simulink model "longSimworks"  (R2023a)
settings: Solver=VariableStepAuto  StartTime=0.0  StopTime=30  RelTol=1e-3
settings Model: Creator=User  LastModifiedBy=User

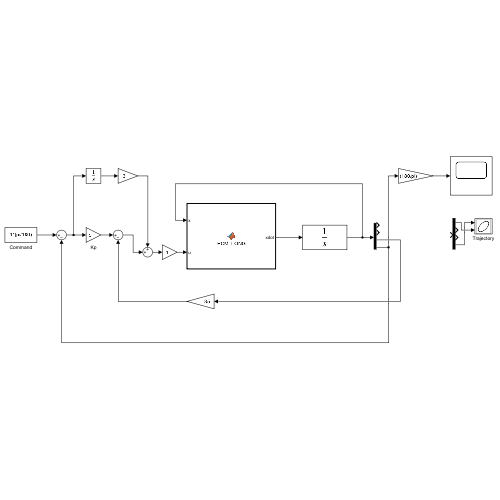
[thumbnail: Simulink's stored preview of the top-level diagram]
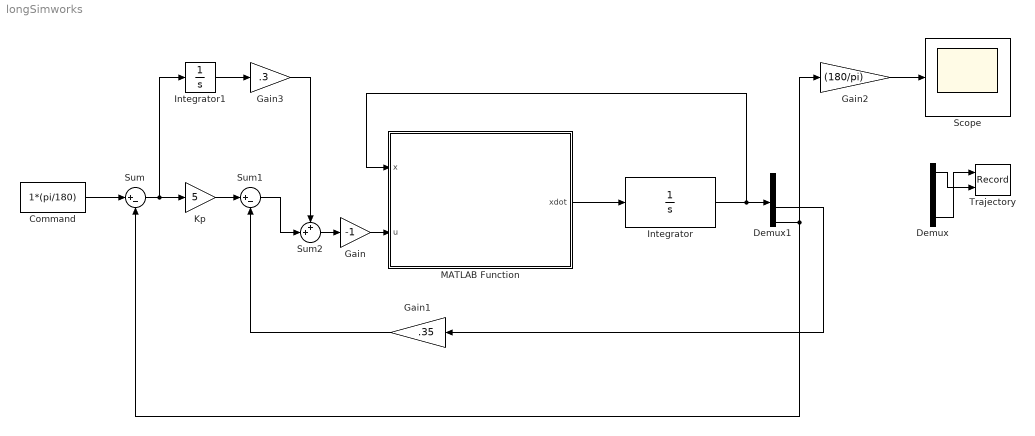
== system longSimworks ==
  Command : Constant  Value=1*(pi/180)
  Demux : Demux
  Demux1 : Demux
  Gain : Gain  Gain=-1
  Gain1 : Gain  Gain=.35
  Gain2 : Gain  Gain=(180/pi)
  Gain3 : Gain  Gain=.3
  Integrator : Integrator  InitialCondition=[0; 0; 0; 0]
  Integrator1 : Integrator
  Kp : Gain  Gain=5
  MATLAB Function : MATLAB Function  TreatAsAtomicUnit=on
  Scope : Scope
  Sum : Sum  Inputs=|+-
  Sum1 : Sum  Inputs=|+-
  Sum2 : Sum  Inputs=++|
  Trajectory : Record  FileSettingsInternal="{\"entries\":[{\"content\":{\"excelSettings\":{\"content\":{},\"type\":\"Streamout.ExcelSettings\"}},\"type\":\"Streamout.FileSettingStorage\",\"uuid\":\"55440844-dddf-4c7d-848c-ec0167b170e0\"}],\"packageUris\":[\"http://schema.mathworks.com/mf0/streamout_blocks/R2020a\"],\"version\":\"1.0\"}"  Layout=[1 2]  SignalsInternal="{\"entries\":[{\"content\":{\"signals\":[{\"content\":{\"blockPath\":[\"longSimworks/Trajectory\"],\"dimensions\":[1],\"domain\":\"longSimworks/Trajectory\",\"lineColor\":\"#a2142f\",\"plots\":[1],\"port\":1,\"sid\":[\"\"],\"signalID\":205,\"signalName\":\"Demux:4\"},\"type\":\"RecordBlkView.Signal\",\"uuid\":\"3001cd2d-3298-47da-9ba3-97cff598d7e7\"},{\"content\":{\"blockPath\":[\"longSimworks/Trajectory\"],\"dimensions\":[1],\"domain\":\"longSimworks/Trajectory\",\"lineColor\":\"#139fff\",\"plots\":[1],\"port\":2,\"sid\":[\"\"],\"signalID\":209,\"signalName\":\"Demux:1\"},\"type\":\"RecordBlkView.Signal\",\"uuid\":\"4ad3851c-6638-45fa-91bf-016d3b368ff9\"}]},\"type\":\"RecordBlkView.InputSignals\",\"uuid\":\"22cb853c-d4ca-4618-9435-a412375c21c1\"}],\"packageUris\":[\"http://schema.mathworks.com/mf0/streamout_blocks/R2020a\"],\"version\":\"1.0\"}"  VisualizationBindings="{\"xyplotplugin\":{\"info\":[{\"series\":[],\"subplotID\":1}]}}"  CompatibilityTag=XY
  wires:
  Sum/1 -> Integrator1/1, Kp/1
  Command/1 -> Sum/1
  Demux/4 -> Trajectory/1
  Demux/1 -> Trajectory/2
  MATLAB Function/1(xdot) -> Integrator/1
  Demux1/3 -> Gain1/1
  Gain1/1 -> Sum1/2
  Kp/1 -> Sum1/1
  Sum1/1 -> Sum2/2
  Integrator/1 -> MATLAB Function/1(x), Demux1/1
  Demux1/4 -> Gain2/1, Sum/2
  Gain2/1 -> Scope/1
  Gain3/1 -> Sum2/1
  Sum2/1 -> Gain/1
  Gain/1 -> MATLAB Function/2(u)
  Integrator1/1 -> Gain3/1

== matlab function longSimworks/MATLAB Function ==
  data: x input; xdot output; u input
function xdot = EOM_LONG(x, u)

%% Initial Mass & Geometry Properties
%Givens
W = 6360; %lb
g = 32.2; %ft/s2
Ixx = 7.99e3; %slug ft2
Iyy = 3.33e3; %slug ft2
Izz = 1.12e4; %slug ft2
Ixz = -3.91e1; %slug ft2

m = W/32.2; %lb

%Inertial Matrix
I = [Ixx, 0,-Ixz;
      0, Iyy, 0;
    -Ixz, 0, Izz]; 

S = 182; %ft2
b = 33.8; %ft
c_hat = 5.47; %ft
x_cg = 27; 
trim_aoa = 0.7; %deg

%% Longitudinal Derivatives
Xu = -0.0168;
Xa = 14.8205;
Zu = -0.1844;
Za = -645.1571;
Mu = 0;
Ma = -28.9722;
Madot = -2.2569;
Mq = -4.8604;
Xde = 0;
Zde = -53.4070;
Mde = -46.4075;
theta = trim_aoa*(pi/180);
U1 = 349;

%% Mapping Out Longitudinal Motion
%unpack state from the q state column vector
x = x(1:4);

%******** Motion *************
A1 = [        Xu                 Xa                   0         -g*cos(theta);
            Zu/U1               Za/U1                1        (-g*sin(theta)/U1);
      Mu + (Madot/U1)*Zu  Ma + Madot*(Za/U1)     Mq + Madot         0;
             0                  0                    1              0];


%******** Control *************
B1 = [    Xde;
         Zde/U1;
      Mde + (Madot/U1)*Zde;
           0];

xdot = A1*x + B1*u;
end
